simulink model "Bai06_2"  (R2023b)
settings: Solver=VariableStepAuto  StartTime=0.0  StopTime=0.1  RelTol=1e-3
settings Model: Creator=Trung  LastModifiedBy=Trung

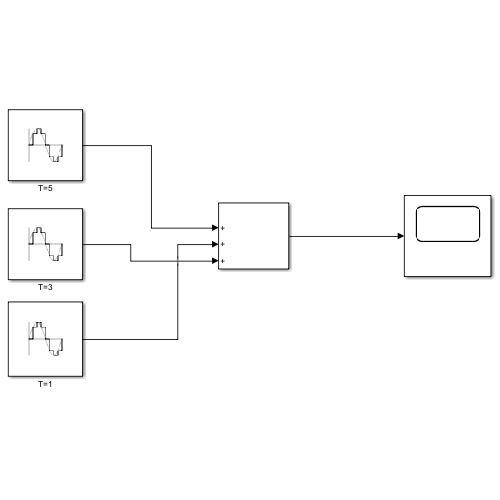
[thumbnail: Simulink's stored preview of the top-level diagram]
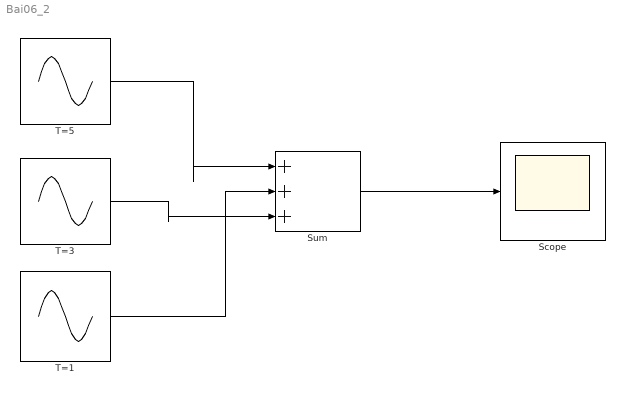
== system Bai06_2 ==
  Scope : Scope
  Sum : Sum  Inputs=|+++
  T=1 : Sin  Frequency=50 * pi * 2  SampleTime=0.0001
  T=3 : Sin  Amplitude=1/3  Frequency=50*pi*2*3  SampleTime=0.0001
  T=5 : Sin  Amplitude=1/5  Frequency=50*pi*2*5  SampleTime=0.0001
  wires:
  T=1/1 -> Sum/2
  T=3/1 -> Sum/3
  Sum/1 -> Scope/1
  T=5/1 -> Sum/1
